simulink model "Properties_Tank1_Primitives"  (R2012b)
settings: Solver=FixedStepDiscrete  StartTime=0.0  StopTime=10.0  FixedStep=0.1  RelTol=1e-3
settings Model: Creator=Kerianne  LastModifiedBy=Kerianne
settings DataIOCC: SaveFormat=Structure
settings OptimizationCC: InlineParams=on

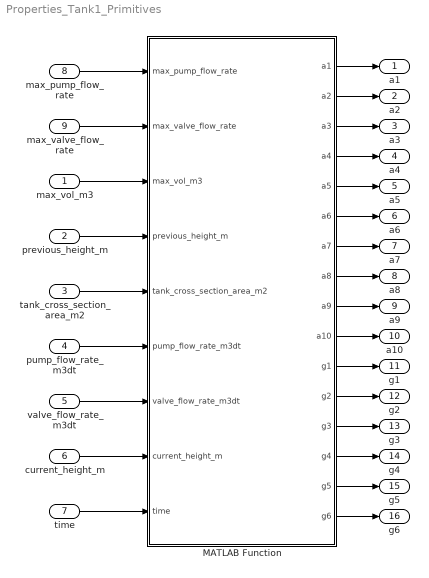
== system Properties_Tank1_Primitives ==
  max_vol_m3 : Inport  OutDataTypeStr=double
  previous_height_m : Inport  Port=2  OutDataTypeStr=double
  tank_cross_section_area_m2 : Inport  Port=3  OutDataTypeStr=double
  pump_flow_rate_m3dt : Inport  Port=4  OutDataTypeStr=double
  valve_flow_rate_m3dt : Inport  Port=5  OutDataTypeStr=double
  current_height_m : Inport  Port=6  OutDataTypeStr=double
  time : Inport  Port=7  OutDataTypeStr=double
  max_pump_flow_rate : Inport  Port=8  OutDataTypeStr=double
  max_valve_flow_rate : Inport  Port=9  OutDataTypeStr=double
  MATLAB Function : MATLAB Function  TreatAsAtomicUnit=on
  a1 : Outport  OutDataTypeStr=boolean
  a2 : Outport  Port=2  OutDataTypeStr=boolean
  a3 : Outport  Port=3  OutDataTypeStr=boolean
  a4 : Outport  Port=4  OutDataTypeStr=boolean
  a5 : Outport  Port=5  OutDataTypeStr=boolean
  a6 : Outport  Port=6  OutDataTypeStr=boolean
  a7 : Outport  Port=7  OutDataTypeStr=boolean
  a8 : Outport  Port=8  OutDataTypeStr=boolean
  a9 : Outport  Port=9  OutDataTypeStr=boolean
  a10 : Outport  Port=10  OutDataTypeStr=boolean
  g1 : Outport  Port=11  OutDataTypeStr=boolean
  g2 : Outport  Port=12  OutDataTypeStr=boolean
  g3 : Outport  Port=13  OutDataTypeStr=boolean
  g4 : Outport  Port=14  OutDataTypeStr=boolean
  g5 : Outport  Port=15  OutDataTypeStr=boolean
  g6 : Outport  Port=16  OutDataTypeStr=boolean
  wires:
  MATLAB Function/1(a1) -> a1/1
  MATLAB Function/2(a2) -> a2/1
  MATLAB Function/16(g6) -> g6/1
  MATLAB Function/15(g5) -> g5/1
  MATLAB Function/14(g4) -> g4/1
  MATLAB Function/13(g3) -> g3/1
  MATLAB Function/12(g2) -> g2/1
  MATLAB Function/11(g1) -> g1/1
  MATLAB Function/8(a8) -> a8/1
  MATLAB Function/7(a7) -> a7/1
  MATLAB Function/6(a6) -> a6/1
  MATLAB Function/5(a5) -> a5/1
  MATLAB Function/4(a4) -> a4/1
  MATLAB Function/3(a3) -> a3/1
  max_vol_m3/1 -> MATLAB Function/3(max_vol_m3)
  previous_height_m/1 -> MATLAB Function/4(previous_height_m)
  tank_cross_section_area_m2/1 -> MATLAB Function/5(tank_cross_section_area_m2)
  pump_flow_rate_m3dt/1 -> MATLAB Function/6(pump_flow_rate_m3dt)
  valve_flow_rate_m3dt/1 -> MATLAB Function/7(valve_flow_rate_m3dt)
  current_height_m/1 -> MATLAB Function/8(current_height_m)
  time/1 -> MATLAB Function/9(time)
  max_pump_flow_rate/1 -> MATLAB Function/1(max_pump_flow_rate)
  max_valve_flow_rate/1 -> MATLAB Function/2(max_valve_flow_rate)
  MATLAB Function/9(a9) -> a9/1
  MATLAB Function/10(a10) -> a10/1

== matlab function Properties_Tank1_Primitives/MATLAB Function ==
  data: max_pump_flow_rate input; max_valve_flow_rate input; a1 output; a2 output; a3 output; a4 output; a5 output; a6 output; a7 output; a8 output; a9 output; a10 output; max_vol_m3 input; g1 output; previous_height_m input; tank_cross_section_area_m2 input; pump_flow_rate_m3dt input; valve_flow_rate_m3dt input; current_height_m input; time input; g2 output; g3 output; g4 output; g5 output; g6 output
function [a1, a2, a3, a4, a5, a6, a7, a8, a9, a10, g1, g2, g3, g4, g5, g6]   = verification_condition(max_pump_flow_rate, max_valve_flow_rate, max_vol_m3, previous_height_m, tank_cross_section_area_m2, pump_flow_rate_m3dt, valve_flow_rate_m3dt, current_height_m, time)

persistent pre_tank_cross_section_area_m2
if isempty(pre_tank_cross_section_area_m2)
    pre_tank_cross_section_area_m2 = tank_cross_section_area_m2;
end
persistent pre_max_vol_m3
if isempty(pre_max_vol_m3)
    pre_max_vol_m3 = max_vol_m3;
end
% Updated 26 Feb 2015 based on tank1.aadl from 20150205

current_volume_m3 = current_height_m*tank_cross_section_area_m2;
previous_volume_m3 = previous_height_m*tank_cross_section_area_m2;
net_flow_m3dt = pump_flow_rate_m3dt - valve_flow_rate_m3dt;
tank_height_m = max_vol_m3/tank_cross_section_area_m2;

% Assumptions
% assume "Pump flow rate is positive"
a1 = pump_flow_rate_m3dt >= 0.0;
% assume "Pump flow rate is initially 0"
a2 = pump_init_no_flow(pump_flow_rate_m3dt, time);
% assume "Tank cross section area is positive"
a3 = tank_cross_section_area_m2 > 0.0;
% assume "Tank cross section area is constant"
a4 = pre_tank_cross_section_area_m2 == tank_cross_section_area_m2;
% assume "Valve flow rate is positive"
a5 = valve_flow_rate_m3dt >= 0.0;
% assume "Tank volume is positive"
a6 = max_vol_m3 >= 0;
% assume "Tank volume is constant"
a7 = pre_max_vol_m3 == max_vol_m3;
% assume "Initial Height of the liquid is 0.0"
a8 = init_0_vol(previous_height_m, time);
% assume valve_flow_rate is 0 or max flow rate
a9 = valve_flow_rate_m3dt == 0.0 | valve_flow_rate_m3dt == max_valve_flow_rate;
% assume pump flow rate is 0 or max flow rate
a10 = pump_flow_rate_m3dt == 0.0 | pump_flow_rate_m3dt == max_pump_flow_rate;



% Guarantees
% guarantee "The initial volume of tank 1 should be equivalent to the specified initial tank 1 volume"
g1 = pump_initially_off(previous_height_m,time,tank_cross_section_area_m2);
% guarantee "If the current tank 1 volume plus the tank 1 net flow is greater than the tank 1 maximum volume then tank 1 is full"
g2 = full_cond(current_volume_m3, previous_volume_m3, net_flow_m3dt, max_vol_m3);
% guarantee "If the current tank 1 volume plus the tank 1 net flow is less than the tank 1 minimum volume then tank 1 is empty" 
g3 = empty_cond(current_volume_m3, previous_volume_m3, net_flow_m3dt);
% guarantee "If the current tank 1 volume plus the tank 1 net flow is greater than empty and less than the tank 1 maximum volume then the tank 1 volume changes by the tank 1 net flow":
g4 = tank_volume_update(current_volume_m3, net_flow_m3dt, max_vol_m3, previous_volume_m3);
% guarantee "Current height of tank 1 is equal or less than the max tank 1 height" 
g5 = tank_less_or_equal_full(current_height_m, tank_height_m);
% guarantee "Current height of tank 1 is non negative" 
g6 = tank_height_not_negative(current_height_m);

pre_max_vol_m3 = max_vol_m3;
pre_tank_cross_section_area_m2 = tank_cross_section_area_m2;

% a2
function result = pump_init_no_flow(pump_flow_rate_m3dt, time)
    UnderThisCondition = (time == 0.0);
    ResultShouldBe = (pump_flow_rate_m3dt == 0.0);
    result = implies(UnderThisCondition, ResultShouldBe);
function result = init_0_vol(previous_height_m, time)
    UnderThisCondition = (time == 0.0);
    ResultShouldBe = (previous_height_m == 0.0);
    result = implies(UnderThisCondition, ResultShouldBe);
function c = implies(a,b)      
     c = ((not (a)) || b);
% g1 "The initial volume of tank 1 should be equivalent to the specified initial tank 1 volume"
function result = pump_initially_off( previous_height_m, time, tank_cross_section_area_m2)
    UnderThisCondition = (time == 0.0);
    ResultShouldBe = (previous_height_m*tank_cross_section_area_m2 == 0.0*tank_cross_section_area_m2);
    result = implies(UnderThisCondition, ResultShouldBe);
% g2 guarantee "If the current tank 1 volume plus the tank 1 net flow is greater than the tank 1 maximum volume then tank 1 is full"
function result = full_cond(current_volume_m3, previous_volume_m3, net_flow_m3dt, max_vol_m3)
    UnderThisCondition = (previous_volume_m3 + net_flow_m3dt >= max_vol_m3);
    ResultShouldBe = (current_volume_m3 == max_vol_m3);
    result = implies(UnderThisCondition, ResultShouldBe);
% g3 "If the current tank 1 volume plus the tank 1 net flow is less than the tank 1 minimum volume then tank 1 is empty"
function result = empty_cond(current_volume_m3, previous_volume_m3, net_flow_m3dt) 
    UnderThisCondition = (previous_volume_m3 + net_flow_m3dt <= 0.0);
    ResultShouldBe = (current_volume_m3 == 0.0);
    result = implies(UnderThisCondition, ResultShouldBe);
% g4 "If the current tank 1 volume plus the tank 1 net flow is greater than empty and less than the tank 1 maximum volume then the tank 1 volume changes by the tank 1 net flow"
function result = tank_volume_update(current_volume_m3, net_flow_m3dt, max_vol_m3, previous_volume_m3)   
    UnderThisCondition = ((previous_volume_m3 + net_flow_m3dt < max_vol_m3) && (previous_volume_m3 + net_flow_m3dt >= 0.0));
    ResultShouldBe = (current_volume_m3 == previous_volume_m3 + net_flow_m3dt);
    result = implies(UnderThisCondition, ResultShouldBe);
% g5 "Current height of tank 1 is equal or less than the max tank 1 height" 
function result = tank_less_or_equal_full(current_height_m, tank_height_m)   
    result = (current_height_m <= tank_height_m);
% g6 "Current height of tank 1 is non negative" 
function result = tank_height_not_negative(current_height_m)   
    result = (current_height_m >= 0);
